simulink model "SCR_SiLS"  (R2021b)
settings: Solver=FixedStepDiscrete  StartTime=0.0  StopTime=inf  FixedStep=0.001  RelTol=1e-3
model workspace (MAT data in the model file):
  DataSet : object (value not decoded)
  DebugLevel = 0
  GuiObj = 0
  GuiObjTemp = 0
  GuiPrefs : object (value not decoded)
  M1TargetParameters : object (value not decoded)
  NbrOfParams = 3
  NbrOfRem = 0
  save_DataSet : object (value not decoded)
  save_NbrOfParams = 3
  save_NbrOfRem = 0
undefined symbols (not defined in the file or in its folder): AI_Test1, AO_Test1, NONOXR4, PLC_PRG, var1_INT16_LREAL_scalar_bus_200_mixed_aligned_out, X20I0Mat_typ, X20IOMat, X20IOSim
libraries: bur_blks x62, M1SWBlocks x8
(part 2 of 2)

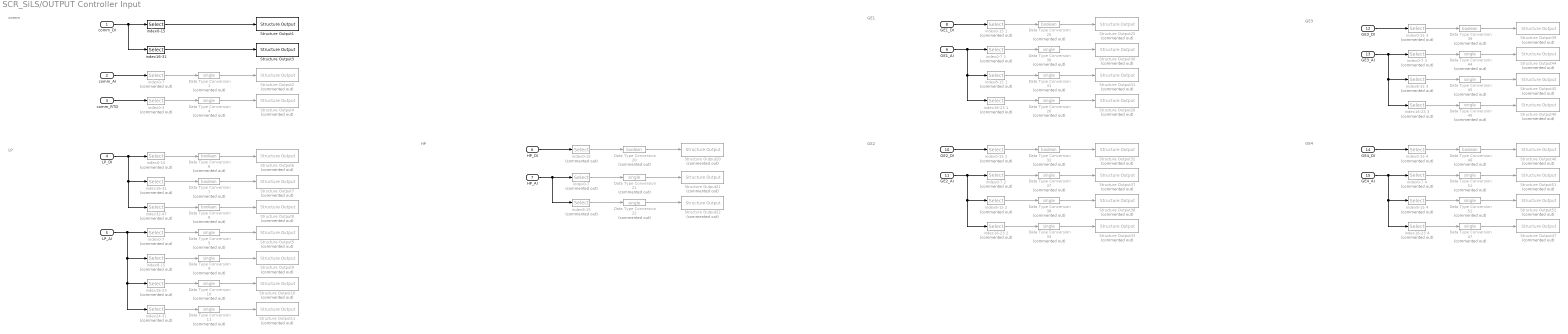
== system SCR_SiLS/OUTPUT Controller Input ==
  note: GE4
  note: GE3
  note: GE2
  note: GE1
  note: HP
  note: LP
  note: comm
  comm_DI : Inport
  comm_AI : Inport  Port=2
  comm_RTD : Inport  Port=3
  LP_DI : Inport  Port=4
  LP_AI : Inport  Port=5
  HP_DI : Inport  Port=6
  HP_AI : Inport  Port=7
  GE1_DI : Inport  Port=8
  GE1_AI : Inport  Port=9
  GE2_DI : Inport  Port=10
  GE2_AI : Inport  Port=11
  GE3_DI : Inport  Port=12
  GE3_AI : Inport  Port=13
  GE4_DI : Inport  Port=14
  GE4_AI : Inport  Port=15
  " index0-15 " : Selector  Commented=on  IndexMode=Zero-based  InputPortWidth=48  IndexOptions=Index vector (dialog)  Indices=[0:15]  OutputSizes=1
  " index0-15 1" : Selector  Commented=on  IndexMode=Zero-based  InputPortWidth=16  IndexOptions=Index vector (dialog)  Indices=[0:15]  OutputSizes=1
  " index0-7 " : Selector  Commented=on  IndexMode=Zero-based  InputPortWidth=32  IndexOptions=Index vector (dialog)  Indices=[0:7]  OutputSizes=1
   index0-7 {1..4} (4 alike) : Selector  Commented=on  IndexMode=Zero-based  InputPortWidth=24  IndexOptions=Index vector (dialog)  Indices=[0:7]  OutputSizes=1
  " index16-23 " : Selector  Commented=on  IndexMode=Zero-based  InputPortWidth=32  IndexOptions=Index vector (dialog)  Indices=[16:23]  OutputSizes=1
   index16-23 {1..4} (4 alike) : Selector  Commented=on  IndexMode=Zero-based  InputPortWidth=24  IndexOptions=Index vector (dialog)  Indices=[16:23]  OutputSizes=1
  " index16-31 " : Selector  Commented=on  IndexMode=Zero-based  InputPortWidth=48  IndexOptions=Index vector (dialog)  Indices=[16:31]  OutputSizes=1
  " index24-31 " : Selector  Commented=on  IndexMode=Zero-based  InputPortWidth=32  IndexOptions=Index vector (dialog)  Indices=[24:31]  OutputSizes=1
  " index32-47 " : Selector  Commented=on  IndexMode=Zero-based  InputPortWidth=48  IndexOptions=Index vector (dialog)  Indices=[32:47]  OutputSizes=1
  " index8-15 " : Selector  Commented=on  IndexMode=Zero-based  InputPortWidth=32  IndexOptions=Index vector (dialog)  Indices=[8:15]  OutputSizes=1
   index8-15 {1..4} (4 alike) : Selector  Commented=on  IndexMode=Zero-based  InputPortWidth=24  IndexOptions=Index vector (dialog)  Indices=[8:15]  OutputSizes=1
  Data Type Conversion{1,4..5,9..11,21..22,26,30..31,33,37..38,40,44..45,47,51..52} (20 alike) : DataTypeConversion  Commented=on  OutDataTypeStr=single
  Data Type Conversion{6..8,20,25,32,39,46} (8 alike) : DataTypeConversion  Commented=on  OutDataTypeStr=boolean
  Structure Output1 : bur_blks/Structure Output  Tag=GLOBAL BOOL X20IOSim.Comm.DIF371[0].Value [0...15]  bur_var_name=X20IOSim.Comm.DIF371[0].Value  bur_scope=GLOBAL  bur_struct_name=X20IOSim  bur_data_type=BOOL  bur_array_index=15  bur_data_type_num=8  bur_AS_string=X20IOSim : X20I0Mat_typ := (0); (**)  bur_struct_reference=X20I0Mat_typ.Comm.DIF371(0).Value  bur_memory=standard
      settings: AttributesFormatString=%<Tag>  SourceProductName=B&R Automation Studio Toolbox
  Structure Output10 : bur_blks/Structure Output  Tag=GLOBAL REAL X20IOSim.LP.AI8321[2].Value [0...7]  Commented=on  bur_var_name=X20IOSim.LP.AI8321[2].Value  bur_scope=GLOBAL  bur_struct_name=X20IOSim  bur_data_type=REAL  bur_array_index=7  bur_data_type_num=1  bur_AS_string=X20IOSim : X20I0Mat_typ := (0); (**)  bur_struct_reference=X20I0Mat_typ.LP.AI8321(2).Value  bur_memory=standard
      settings: AttributesFormatString=%<Tag>  SourceProductName=B&R Automation Studio Toolbox
  Structure Output11 : bur_blks/Structure Output  Tag=GLOBAL REAL X20IOSim.LP.AI8321[3].Value [0...7]  Commented=on  bur_var_name=X20IOSim.LP.AI8321[3].Value  bur_scope=GLOBAL  bur_struct_name=X20IOSim  bur_data_type=REAL  bur_array_index=7  bur_data_type_num=1  bur_AS_string=X20IOSim : X20I0Mat_typ := (0); (**)  bur_struct_reference=X20I0Mat_typ.LP.AI8321(3).Value  bur_memory=standard
      settings: AttributesFormatString=%<Tag>  SourceProductName=B&R Automation Studio Toolbox
  Structure Output2 : bur_blks/Structure Output  Tag=GLOBAL REAL X20IOSim.Comm.AI8321[0].Value [0...7]  Commented=on  bur_var_name=X20IOSim.Comm.AI8321[0].Value  bur_scope=GLOBAL  bur_struct_name=X20IOSim  bur_data_type=REAL  bur_array_index=7  bur_data_type_num=1  bur_AS_string=X20IOSim : X20I0Mat_typ := (0); (**)  bur_struct_reference=X20I0Mat_typ.Comm.AI8321(0).Value  bur_memory=standard
      settings: AttributesFormatString=%<Tag>  SourceProductName=B&R Automation Studio Toolbox
  Structure Output20 : bur_blks/Structure Output  Tag=GLOBAL BOOL X20IOSim.HP.DIF371[0].Value [0...15]  Commented=on  bur_var_name=X20IOSim.HP.DIF371[0].Value  bur_scope=GLOBAL  bur_struct_name=X20IOSim  bur_data_type=BOOL  bur_array_index=15  bur_data_type_num=8  bur_AS_string=X20IOSim : X20I0Mat_typ := (0); (**)  bur_struct_reference=X20I0Mat_typ.HP.DIF371(0).Value  bur_memory=standard
      settings: AttributesFormatString=%<Tag>  SourceProductName=B&R Automation Studio Toolbox
  Structure Output21 : bur_blks/Structure Output  Tag=GLOBAL REAL X20IOSim.HP.AI8321[0].Value [0...7]  Commented=on  bur_var_name=X20IOSim.HP.AI8321[0].Value  bur_scope=GLOBAL  bur_struct_name=X20IOSim  bur_data_type=REAL  bur_array_index=7  bur_data_type_num=1  bur_AS_string=X20IOSim : X20I0Mat_typ := (0); (**)  bur_struct_reference=X20I0Mat_typ.HP.AI8321(0).Value  bur_memory=standard
      settings: AttributesFormatString=%<Tag>  SourceProductName=B&R Automation Studio Toolbox
  Structure Output22 : bur_blks/Structure Output  Tag=GLOBAL REAL X20IOSim.HP.AI8321[1].Value [0...7]  Commented=on  bur_var_name=X20IOSim.HP.AI8321[1].Value  bur_scope=GLOBAL  bur_struct_name=X20IOSim  bur_data_type=REAL  bur_array_index=7  bur_data_type_num=1  bur_AS_string=X20IOSim : X20I0Mat_typ := (0); (**)  bur_struct_reference=X20I0Mat_typ.HP.AI8321(1).Value  bur_memory=standard
      settings: AttributesFormatString=%<Tag>  SourceProductName=B&R Automation Studio Toolbox
  Structure Output25 : bur_blks/Structure Output  Tag=GLOBAL BOOL X20IOSim.GE1.DIF371[0].Value [0...15]  Commented=on  bur_var_name=X20IOSim.GE1.DIF371[0].Value  bur_scope=GLOBAL  bur_struct_name=X20IOSim  bur_data_type=BOOL  bur_array_index=15  bur_data_type_num=8  bur_AS_string=X20IOSim : X20I0Mat_typ := (0); (**)  bur_struct_reference=X20I0Mat_typ.GE1.DIF371(0).Value  bur_memory=standard
      settings: AttributesFormatString=%<Tag>  SourceProductName=B&R Automation Studio Toolbox
  Structure Output26 : bur_blks/Structure Output  Tag=GLOBAL REAL X20IOSim.GE1.AI8321[2].Value [0...7]  Commented=on  bur_var_name=X20IOSim.GE1.AI8321[2].Value  bur_scope=GLOBAL  bur_struct_name=X20IOSim  bur_data_type=REAL  bur_array_index=7  bur_data_type_num=1  bur_AS_string=X20IOSim : X20I0Mat_typ := (0); (**)  bur_struct_reference=X20I0Mat_typ.GE1.AI8321(2).Value  bur_memory=standard
      settings: AttributesFormatString=%<Tag>  SourceProductName=B&R Automation Studio Toolbox
  Structure Output3 : bur_blks/Structure Output  Tag=GLOBAL BOOL X20IOSim.Comm.DIF371[1].Value [0...15]  bur_var_name=X20IOSim.Comm.DIF371[1].Value  bur_scope=GLOBAL  bur_struct_name=X20IOSim  bur_data_type=BOOL  bur_array_index=15  bur_data_type_num=8  bur_AS_string=X20IOSim : X20I0Mat_typ := (0); (**)  bur_struct_reference=X20I0Mat_typ.Comm.DIF371(1).Value  bur_memory=standard
      settings: AttributesFormatString=%<Tag>  SourceProductName=B&R Automation Studio Toolbox
  Structure Output30 : bur_blks/Structure Output  Tag=GLOBAL REAL X20IOSim.GE1.AI8321[0].Value [0...7]  Commented=on  bur_var_name=X20IOSim.GE1.AI8321[0].Value  bur_scope=GLOBAL  bur_struct_name=X20IOSim  bur_data_type=REAL  bur_array_index=7  bur_data_type_num=1  bur_AS_string=X20IOSim : X20I0Mat_typ := (0); (**)  bur_struct_reference=X20I0Mat_typ.GE1.AI8321(0).Value  bur_memory=standard
      settings: AttributesFormatString=%<Tag>  SourceProductName=B&R Automation Studio Toolbox
  Structure Output31 : bur_blks/Structure Output  Tag=GLOBAL REAL X20IOSim.GE1.AI8321[1].Value [0...7]  Commented=on  bur_var_name=X20IOSim.GE1.AI8321[1].Value  bur_scope=GLOBAL  bur_struct_name=X20IOSim  bur_data_type=REAL  bur_array_index=7  bur_data_type_num=1  bur_AS_string=X20IOSim : X20I0Mat_typ := (0); (**)  bur_struct_reference=X20I0Mat_typ.GE1.AI8321(1).Value  bur_memory=standard
      settings: AttributesFormatString=%<Tag>  SourceProductName=B&R Automation Studio Toolbox
  Structure Output32 : bur_blks/Structure Output  Tag=GLOBAL BOOL X20IOSim.GE2.DIF371[0].Value [0...15]  Commented=on  bur_var_name=X20IOSim.GE2.DIF371[0].Value  bur_scope=GLOBAL  bur_struct_name=X20IOSim  bur_data_type=BOOL  bur_array_index=15  bur_data_type_num=8  bur_AS_string=X20IOSim : X20I0Mat_typ := (0); (**)  bur_struct_reference=X20I0Mat_typ.GE2.DIF371(0).Value  bur_memory=standard
      settings: AttributesFormatString=%<Tag>  SourceProductName=B&R Automation Studio Toolbox
  Structure Output33 : bur_blks/Structure Output  Tag=GLOBAL REAL X20IOSim.GE2.AI8321[2].Value [0...7]  Commented=on  bur_var_name=X20IOSim.GE2.AI8321[2].Value  bur_scope=GLOBAL  bur_struct_name=X20IOSim  bur_data_type=REAL  bur_array_index=7  bur_data_type_num=1  bur_AS_string=X20IOSim : X20I0Mat_typ := (0); (**)  bur_struct_reference=X20I0Mat_typ.GE2.AI8321(2).Value  bur_memory=standard
      settings: AttributesFormatString=%<Tag>  SourceProductName=B&R Automation Studio Toolbox
  Structure Output37 : bur_blks/Structure Output  Tag=GLOBAL REAL X20IOSim.GE2.AI8321[0].Value [0...7]  Commented=on  bur_var_name=X20IOSim.GE2.AI8321[0].Value  bur_scope=GLOBAL  bur_struct_name=X20IOSim  bur_data_type=REAL  bur_array_index=7  bur_data_type_num=1  bur_AS_string=X20IOSim : X20I0Mat_typ := (0); (**)  bur_struct_reference=X20I0Mat_typ.GE2.AI8321(0).Value  bur_memory=standard
      settings: AttributesFormatString=%<Tag>  SourceProductName=B&R Automation Studio Toolbox
  Structure Output38 : bur_blks/Structure Output  Tag=GLOBAL REAL X20IOSim.GE2.AI8321[1].Value [0...7]  Commented=on  bur_var_name=X20IOSim.GE2.AI8321[1].Value  bur_scope=GLOBAL  bur_struct_name=X20IOSim  bur_data_type=REAL  bur_array_index=7  bur_data_type_num=1  bur_AS_string=X20IOSim : X20I0Mat_typ := (0); (**)  bur_struct_reference=X20I0Mat_typ.GE2.AI8321(1).Value  bur_memory=standard
      settings: AttributesFormatString=%<Tag>  SourceProductName=B&R Automation Studio Toolbox
  Structure Output39 : bur_blks/Structure Output  Tag=GLOBAL BOOL X20IOSim.GE3.DIF371[0].Value [0...15]  Commented=on  bur_var_name=X20IOSim.GE3.DIF371[0].Value  bur_scope=GLOBAL  bur_struct_name=X20IOSim  bur_data_type=BOOL  bur_array_index=15  bur_data_type_num=8  bur_AS_string=X20IOSim : X20I0Mat_typ := (0); (**)  bur_struct_reference=X20I0Mat_typ.GE3.DIF371(0).Value  bur_memory=standard
      settings: AttributesFormatString=%<Tag>  SourceProductName=B&R Automation Studio Toolbox
  Structure Output4 : bur_blks/Structure Output  Tag=GLOBAL REAL X20IOSim.Comm.AI4222[0].Value [0...3]  Commented=on  bur_var_name=X20IOSim.Comm.AI4222[0].Value  bur_scope=GLOBAL  bur_struct_name=X20IOSim  bur_data_type=REAL  bur_array_index=3  bur_data_type_num=1  bur_AS_string=X20IOSim : X20I0Mat_typ := (0); (**)  bur_struct_reference=X20I0Mat_typ.Comm.AI4222(0).Value  bur_memory=standard
      settings: AttributesFormatString=%<Tag>  SourceProductName=B&R Automation Studio Toolbox
  Structure Output40 : bur_blks/Structure Output  Tag=GLOBAL REAL X20IOSim.GE3.AI8321[2].Value [0...7]  Commented=on  bur_var_name=X20IOSim.GE3.AI8321[2].Value  bur_scope=GLOBAL  bur_struct_name=X20IOSim  bur_data_type=REAL  bur_array_index=7  bur_data_type_num=1  bur_AS_string=X20IOSim : X20I0Mat_typ := (0); (**)  bur_struct_reference=X20I0Mat_typ.GE3.AI8321(2).Value  bur_memory=standard
      settings: AttributesFormatString=%<Tag>  SourceProductName=B&R Automation Studio Toolbox
  Structure Output44 : bur_blks/Structure Output  Tag=GLOBAL REAL X20IOMat.GE3.AI8321[0].Value [0...7]  Commented=on  bur_var_name=X20IOMat.GE3.AI8321[0].Value  bur_scope=GLOBAL  bur_struct_name=X20IOMat  bur_data_type=REAL  bur_array_index=7  bur_data_type_num=1  bur_AS_string=X20IOMat : X20I0Mat_typ := (0); (**)  bur_struct_reference=X20I0Mat_typ.GE3.AI8321(0).Value  bur_memory=standard
      settings: AttributesFormatString=%<Tag>  SourceProductName=B&R Automation Studio Toolbox
  Structure Output45 : bur_blks/Structure Output  Tag=GLOBAL REAL X20IOSim.GE3.AI8321[1].Value [0...7]  Commented=on  bur_var_name=X20IOSim.GE3.AI8321[1].Value  bur_scope=GLOBAL  bur_struct_name=X20IOSim  bur_data_type=REAL  bur_array_index=7  bur_data_type_num=1  bur_AS_string=X20IOSim : X20I0Mat_typ := (0); (**)  bur_struct_reference=X20I0Mat_typ.GE3.AI8321(1).Value  bur_memory=standard
      settings: AttributesFormatString=%<Tag>  SourceProductName=B&R Automation Studio Toolbox
  Structure Output46 : bur_blks/Structure Output  Tag=GLOBAL BOOL X20IOSim.GE4.DIF371[0].Value [0...15]  Commented=on  bur_var_name=X20IOSim.GE4.DIF371[0].Value  bur_scope=GLOBAL  bur_struct_name=X20IOSim  bur_data_type=BOOL  bur_array_index=15  bur_data_type_num=8  bur_AS_string=X20IOSim : X20I0Mat_typ := (0); (**)  bur_struct_reference=X20I0Mat_typ.GE4.DIF371(0).Value  bur_memory=standard
      settings: AttributesFormatString=%<Tag>  SourceProductName=B&R Automation Studio Toolbox
  Structure Output47 : bur_blks/Structure Output  Tag=GLOBAL REAL X20IOMat.GE4.AI8321[2].Value [0...7]  Commented=on  bur_var_name=X20IOMat.GE4.AI8321[2].Value  bur_scope=GLOBAL  bur_struct_name=X20IOMat  bur_data_type=REAL  bur_array_index=7  bur_data_type_num=1  bur_AS_string=X20IOMat : X20I0Mat_typ := (0); (**)  bur_struct_reference=X20I0Mat_typ.GE4.AI8321(2).Value  bur_memory=standard
      settings: AttributesFormatString=%<Tag>  SourceProductName=B&R Automation Studio Toolbox
  Structure Output5 : bur_blks/Structure Output  Tag=GLOBAL REAL X20IOSim.LP.AI8321[0].Value [0...7]  Commented=on  bur_var_name=X20IOSim.LP.AI8321[0].Value  bur_scope=GLOBAL  bur_struct_name=X20IOSim  bur_data_type=REAL  bur_array_index=7  bur_data_type_num=1  bur_AS_string=X20IOSim : X20I0Mat_typ := (0); (**)  bur_struct_reference=X20I0Mat_typ.LP.AI8321(0).Value  bur_memory=standard
      settings: AttributesFormatString=%<Tag>  SourceProductName=B&R Automation Studio Toolbox
  Structure Output51 : bur_blks/Structure Output  Tag=GLOBAL REAL X20IOSim.GE4.AI8321[0].Value [0...7]  Commented=on  bur_var_name=X20IOSim.GE4.AI8321[0].Value  bur_scope=GLOBAL  bur_struct_name=X20IOSim  bur_data_type=REAL  bur_array_index=7  bur_data_type_num=1  bur_AS_string=X20IOSim : X20I0Mat_typ := (0); (**)  bur_struct_reference=X20I0Mat_typ.GE4.AI8321(0).Value  bur_memory=standard
      settings: AttributesFormatString=%<Tag>  SourceProductName=B&R Automation Studio Toolbox
  Structure Output52 : bur_blks/Structure Output  Tag=GLOBAL REAL X20IOMat.GE4.AI8321[1].Value [0...7]  Commented=on  bur_var_name=X20IOMat.GE4.AI8321[1].Value  bur_scope=GLOBAL  bur_struct_name=X20IOMat  bur_data_type=REAL  bur_array_index=7  bur_data_type_num=1  bur_AS_string=X20IOMat : X20I0Mat_typ := (0); (**)  bur_struct_reference=X20I0Mat_typ.GE4.AI8321(1).Value  bur_memory=standard
      settings: AttributesFormatString=%<Tag>  SourceProductName=B&R Automation Studio Toolbox
  Structure Output6 : bur_blks/Structure Output  Tag=GLOBAL BOOL X20IOSim.LP.DIF371[0].Value [0...15]  Commented=on  bur_var_name=X20IOSim.LP.DIF371[0].Value  bur_scope=GLOBAL  bur_struct_name=X20IOSim  bur_data_type=BOOL  bur_array_index=15  bur_data_type_num=8  bur_AS_string=X20IOSim : X20I0Mat_typ := (0); (**)  bur_struct_reference=X20I0Mat_typ.LP.DIF371(0).Value  bur_memory=standard
      settings: AttributesFormatString=%<Tag>  SourceProductName=B&R Automation Studio Toolbox
  Structure Output7 : bur_blks/Structure Output  Tag=GLOBAL BOOL X20IOSim.LP.DIF371[1].Value [0...15]  Commented=on  bur_var_name=X20IOSim.LP.DIF371[1].Value  bur_scope=GLOBAL  bur_struct_name=X20IOSim  bur_data_type=BOOL  bur_array_index=15  bur_data_type_num=8  bur_AS_string=X20IOSim : X20I0Mat_typ := (0); (**)  bur_struct_reference=X20I0Mat_typ.LP.DIF371(1).Value  bur_memory=standard
      settings: AttributesFormatString=%<Tag>  SourceProductName=B&R Automation Studio Toolbox
  Structure Output8 : bur_blks/Structure Output  Tag=GLOBAL BOOL X20IOSim.LP.DIF371[2].Value [0...15]  Commented=on  bur_var_name=X20IOSim.LP.DIF371[2].Value  bur_scope=GLOBAL  bur_struct_name=X20IOSim  bur_data_type=BOOL  bur_array_index=15  bur_data_type_num=8  bur_AS_string=X20IOSim : X20I0Mat_typ := (0); (**)  bur_struct_reference=X20I0Mat_typ.LP.DIF371(2).Value  bur_memory=standard
      settings: AttributesFormatString=%<Tag>  SourceProductName=B&R Automation Studio Toolbox
  Structure Output9 : bur_blks/Structure Output  Tag=GLOBAL REAL X20IOSim.LP.AI8321[1].Value [0...7]  Commented=on  bur_var_name=X20IOSim.LP.AI8321[1].Value  bur_scope=GLOBAL  bur_struct_name=X20IOSim  bur_data_type=REAL  bur_array_index=7  bur_data_type_num=1  bur_AS_string=X20IOSim : X20I0Mat_typ := (0); (**)  bur_struct_reference=X20I0Mat_typ.LP.AI8321(1).Value  bur_memory=standard
      settings: AttributesFormatString=%<Tag>  SourceProductName=B&R Automation Studio Toolbox
  index0-15 : Selector  IndexMode=Zero-based  InputPortWidth=32  IndexOptions=Index vector (dialog)  Indices=[0:15]  OutputSizes=1
  index0-15 {,2..4} (4 alike) : Selector  Commented=on  IndexMode=Zero-based  InputPortWidth=16  IndexOptions=Index vector (dialog)  Indices=[0:15]  OutputSizes=1
  index0-3 : Selector  Commented=on  IndexMode=Zero-based  InputPortWidth=4  IndexOptions=Index vector (dialog)  Indices=[0:3]  OutputSizes=1
  index0-7 : Selector  Commented=on  IndexMode=Zero-based  InputPortWidth=8  IndexOptions=Index vector (dialog)  Indices=[0:7]  OutputSizes=1
  "index0-7 " : Selector  Commented=on  IndexMode=Zero-based  InputPortWidth=16  IndexOptions=Index vector (dialog)  Indices=[0:7]  OutputSizes=1
  index16-31 : Selector  IndexMode=Zero-based  InputPortWidth=32  IndexOptions=Index vector (dialog)  Indices=[16:31]  OutputSizes=1
  "index8-15 " : Selector  Commented=on  IndexMode=Zero-based  InputPortWidth=16  IndexOptions=Index vector (dialog)  Indices=[8:15]  OutputSizes=1
  wires:
  comm_DI/1 -> index16-31/1, index0-15/1
  comm_AI/1 -> index0-7/1
  index0-7/1 -> Data Type Conversion1/1
  Data Type Conversion1/1 -> Structure Output2/1
  index0-15/1 -> Structure Output1/1
  index16-31/1 -> Structure Output3/1
  Data Type Conversion7/1 -> Structure Output7/1
  Data Type Conversion6/1 -> Structure Output6/1
  " index16-31 "/1 -> Data Type Conversion7/1
  " index0-15 "/1 -> Data Type Conversion6/1
  LP_DI/1 -> " index32-47 "/1, " index16-31 "/1, " index0-15 "/1
  " index32-47 "/1 -> Data Type Conversion8/1
  Data Type Conversion8/1 -> Structure Output8/1
  " index8-15 "/1 -> Data Type Conversion9/1
  Data Type Conversion9/1 -> Structure Output9/1
  Data Type Conversion5/1 -> Structure Output5/1
  " index0-7 "/1 -> Data Type Conversion5/1
  Data Type Conversion10/1 -> Structure Output10/1
  " index16-23 "/1 -> Data Type Conversion10/1
  " index24-31 "/1 -> Data Type Conversion11/1
  Data Type Conversion11/1 -> Structure Output11/1
  LP_AI/1 -> " index24-31 "/1, " index16-23 "/1, " index8-15 "/1, " index0-7 "/1
  "index0-15 "/1 -> Data Type Conversion20/1
  Data Type Conversion20/1 -> Structure Output20/1
  HP_DI/1 -> "index0-15 "/1
  "index0-7 "/1 -> Data Type Conversion21/1
  Data Type Conversion21/1 -> Structure Output21/1
  Data Type Conversion22/1 -> Structure Output22/1
  "index8-15 "/1 -> Data Type Conversion22/1
  HP_AI/1 -> "index0-7 "/1, "index8-15 "/1
  GE1_DI/1 -> " index0-15 1"/1
  Data Type Conversion25/1 -> Structure Output25/1
  " index0-15 1"/1 -> Data Type Conversion25/1
  Data Type Conversion26/1 -> Structure Output26/1
  " index16-23 1"/1 -> Data Type Conversion26/1
  " index0-7 1"/1 -> Data Type Conversion30/1
  Data Type Conversion31/1 -> Structure Output31/1
  " index8-15 1"/1 -> Data Type Conversion31/1
  GE1_AI/1 -> " index16-23 1"/1, " index8-15 1"/1, " index0-7 1"/1
  Data Type Conversion30/1 -> Structure Output30/1
  Data Type Conversion37/1 -> Structure Output37/1
  GE2_AI/1 -> " index0-7 2"/1, " index8-15 2"/1, " index16-23 2"/1
  " index8-15 2"/1 -> Data Type Conversion38/1
  Data Type Conversion38/1 -> Structure Output38/1
  " index0-7 2"/1 -> Data Type Conversion37/1
  " index16-23 2"/1 -> Data Type Conversion33/1
  Data Type Conversion33/1 -> Structure Output33/1
  index0-15 2/1 -> Data Type Conversion32/1
  Data Type Conversion32/1 -> Structure Output32/1
  GE2_DI/1 -> index0-15 2/1
  GE3_DI/1 -> index0-15 3/1
  Data Type Conversion39/1 -> Structure Output39/1
  Data Type Conversion40/1 -> Structure Output40/1
  Data Type Conversion44/1 -> Structure Output44/1
  " index16-23 3"/1 -> Data Type Conversion40/1
  " index0-7 3"/1 -> Data Type Conversion44/1
  Data Type Conversion45/1 -> Structure Output45/1
  " index8-15 3"/1 -> Data Type Conversion45/1
  GE3_AI/1 -> " index0-7 3"/1, " index8-15 3"/1, " index16-23 3"/1
  index0-15 3/1 -> Data Type Conversion39/1
  index0-15 4/1 -> Data Type Conversion46/1
  GE4_AI/1 -> " index0-7 4"/1, " index8-15 4"/1, " index16-23 4"/1
  " index8-15 4"/1 -> Data Type Conversion52/1
  Data Type Conversion52/1 -> Structure Output52/1
  " index0-7 4"/1 -> Data Type Conversion51/1
  " index16-23 4"/1 -> Data Type Conversion47/1
  Data Type Conversion51/1 -> Structure Output51/1
  Data Type Conversion47/1 -> Structure Output47/1
  Data Type Conversion46/1 -> Structure Output46/1
  GE4_DI/1 -> index0-15 4/1
  Data Type Conversion4/1 -> Structure Output4/1
  index0-3/1 -> Data Type Conversion4/1
  comm_RTD/1 -> index0-3/1

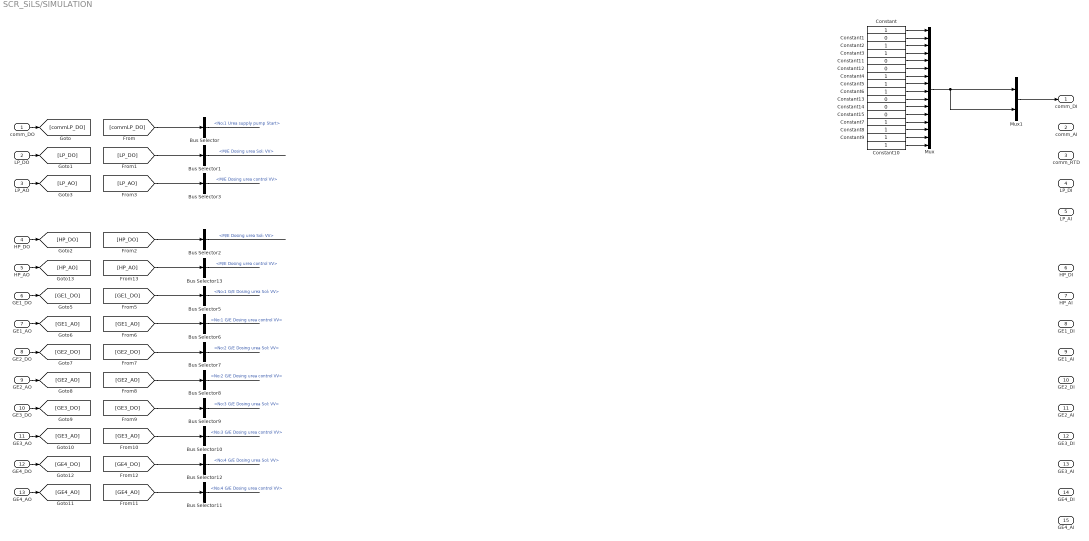
== system SCR_SiLS/SIMULATION ==
  comm_DO : Inport
  LP_DO : Inport  Port=2
  LP_AO : Inport  Port=3
  HP_DO : Inport  Port=4
  HP_AO : Inport  Port=5
  GE1_DO : Inport  Port=6
  GE1_AO : Inport  Port=7
  GE2_DO : Inport  Port=8
  GE2_AO : Inport  Port=9
  GE3_DO : Inport  Port=10
  GE3_AO : Inport  Port=11
  GE4_DO : Inport  Port=12
  GE4_AO : Inport  Port=13
  Bus Selector : BusSelector  OutputSignals=No:1 Urea supply pump Start
  Bus Selector1 : BusSelector  OutputSignals=M/E Dosing urea Sol: VV
  Bus Selector10 : BusSelector  OutputSignals=No:3 G/E Dosing urea control VV
  Bus Selector11 : BusSelector  OutputSignals=No:4 G/E Dosing urea control VV
  Bus Selector12 : BusSelector  OutputSignals=No:4 G/E Dosing urea Sol: VV
  Bus Selector13 : BusSelector  OutputSignals=M/E Dosing urea control VV
  Bus Selector2 : BusSelector  OutputSignals=M/E Dosing urea Sol: VV
  Bus Selector3 : BusSelector  OutputSignals=M/E Dosing urea control VV
  Bus Selector5 : BusSelector  OutputSignals=No:1 G/E Dosing urea Sol: VV
  Bus Selector6 : BusSelector  OutputSignals=No:1 G/E Dosing urea control VV
  Bus Selector7 : BusSelector  OutputSignals=No:2 G/E Dosing urea Sol: VV
  Bus Selector8 : BusSelector  OutputSignals=No:2 G/E Dosing urea control VV
  Bus Selector9 : BusSelector  OutputSignals=No:3 G/E Dosing urea Sol: VV
  Constant{,2..10} (10 alike) : Constant  OutDataTypeStr=boolean
  Constant{1,11..15} (6 alike) : Constant  Value=0  OutDataTypeStr=boolean
  Mux : Mux  Inputs=16
  Mux1 : Mux  Inputs=2
  comm_DI : Outport  VectorParamsAs1DForOutWhenUnconnected=off
  comm_AI : Outport  Port=2  VectorParamsAs1DForOutWhenUnconnected=off
  comm_RTD : Outport  Port=3  VectorParamsAs1DForOutWhenUnconnected=off
  LP_DI : Outport  Port=4  VectorParamsAs1DForOutWhenUnconnected=off
  LP_AI : Outport  Port=5  VectorParamsAs1DForOutWhenUnconnected=off
  HP_DI : Outport  Port=6  VectorParamsAs1DForOutWhenUnconnected=off
  HP_AI : Outport  Port=7  VectorParamsAs1DForOutWhenUnconnected=off
  GE1_DI : Outport  Port=8  VectorParamsAs1DForOutWhenUnconnected=off
  GE1_AI : Outport  Port=9  VectorParamsAs1DForOutWhenUnconnected=off
  GE2_DI : Outport  Port=10  VectorParamsAs1DForOutWhenUnconnected=off
  GE2_AI : Outport  Port=11  VectorParamsAs1DForOutWhenUnconnected=off
  GE3_DI : Outport  Port=12  VectorParamsAs1DForOutWhenUnconnected=off
  GE3_AI : Outport  Port=13  VectorParamsAs1DForOutWhenUnconnected=off
  GE4_DI : Outport  Port=14  VectorParamsAs1DForOutWhenUnconnected=off
  GE4_AI : Outport  Port=15  VectorParamsAs1DForOutWhenUnconnected=off
  wires:
  Bus Selector5/1 -> ?  "<No:1 G/E Dosing urea Sol: VV>"
  Bus Selector3/1 -> ?  "<M/E Dosing urea control VV>"
  Bus Selector/1 -> ?  "<No:1 Urea supply pump Start>"
  Bus Selector8/1 -> ?  "<No:2 G/E Dosing urea control VV>"
  [GE1_AO] -> Bus Selector6/1
  Bus Selector2/1 -> ?  "<M/E Dosing urea Sol: VV>"
  [GE1_DO] -> Bus Selector5/1
  [LP_AO] -> Bus Selector3/1
  [LP_DO] -> Bus Selector1/1
  [commLP_DO] -> Bus Selector/1
  [GE2_DO] -> Bus Selector7/1
  Bus Selector7/1 -> ?  "<No:2 G/E Dosing urea Sol: VV>"
  [HP_DO] -> Bus Selector2/1
  Bus Selector12/1 -> ?  "<No:4 G/E Dosing urea Sol: VV>"
  Bus Selector13/1 -> ?  "<M/E Dosing urea control VV>"
  [GE4_AO] -> Bus Selector11/1
  [GE3_AO] -> Bus Selector10/1
  Bus Selector11/1 -> ?  "<No:4 G/E Dosing urea control VV>"
  [GE4_DO] -> Bus Selector12/1
  [GE2_AO] -> Bus Selector8/1
  [GE3_DO] -> Bus Selector9/1
  Bus Selector9/1 -> ?  "<No:3 G/E Dosing urea Sol: VV>"
  Bus Selector10/1 -> ?  "<No:3 G/E Dosing urea control VV>"
  Bus Selector6/1 -> ?  "<No:1 G/E Dosing urea control VV>"
  Bus Selector1/1 -> ?  "<M/E Dosing urea Sol: VV>"
  [HP_AO] -> Bus Selector13/1
  comm_DO/1 -> [commLP_DO]
  LP_DO/1 -> [LP_DO]
  LP_AO/1 -> [LP_AO]
  HP_DO/1 -> [HP_DO]
  HP_AO/1 -> [HP_AO]
  GE1_DO/1 -> [GE1_DO]
  GE2_DO/1 -> [GE2_DO]
  GE1_AO/1 -> [GE1_AO]
  GE2_AO/1 -> [GE2_AO]
  GE3_DO/1 -> [GE3_DO]
  GE3_AO/1 -> [GE3_AO]
  GE4_DO/1 -> [GE4_DO]
  GE4_AO/1 -> [GE4_AO]
  Mux1/1 -> comm_DI/1
  Constant/1 -> Mux/1
  Constant1/1 -> Mux/2
  Constant2/1 -> Mux/3
  Constant3/1 -> Mux/4
  Constant11/1 -> Mux/5
  Constant12/1 -> Mux/6
  Constant4/1 -> Mux/7
  Constant5/1 -> Mux/8
  Constant6/1 -> Mux/9
  Constant13/1 -> Mux/10
  Constant14/1 -> Mux/11
  Constant15/1 -> Mux/12
  Constant7/1 -> Mux/13
  Constant8/1 -> Mux/14
  Constant9/1 -> Mux/15
  Constant10/1 -> Mux/16
  Mux/1 -> Mux1/2, Mux1/1
